simulink model "no_clock_simulink"  (Simulink 7.8)
settings: Solver=VariableStepDiscrete  StartTime=0.0  StopTime=10.0  RelTol=1e-3
values from neighbouring files (symbols this model uses):
  in24b = uut.v_24bit    [no_clock_index_test.m]    (also in no_clock_test.m = double(uut.in_24bit))
  in64b1 = double(typecast(uut.in_64bit,'uint32'))    [no_clock_test.m]
  in64b2 = 0    [no_clock_test.m]
  in8b = double(uut.in_8bit)    [no_clock_test.m]
  in96b1 = double(typecast(uut.in_96bit(1),'uint32'))    [no_clock_test.m]
  in96b2 = double(typecast(uut.in_96bit(2),'uint32'))    [no_clock_test.m]
  in96b3 = double(typecast(uut.in_96bit(3),'uint32'))    [no_clock_test.m]
settings Model: Creator=chuh  LastModifiedBy=chuh

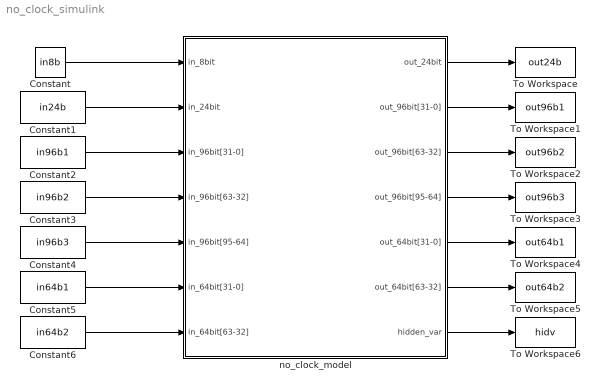
== system no_clock_simulink ==
  Constant : Constant  Value=in8b
  Constant1 : Constant  Value=in24b
  Constant2 : Constant  Value=in96b1
  Constant3 : Constant  Value=in96b2
  Constant4 : Constant  Value=in96b3
  Constant5 : Constant  Value=in64b1
  Constant6 : Constant  Value=in64b2
  To Workspace : ToWorkspace  VariableName=out24b  SampleTime=-1  SaveFormat=Array
  To Workspace1 : ToWorkspace  VariableName=out96b1  SampleTime=-1  SaveFormat=Array
  To Workspace2 : ToWorkspace  VariableName=out96b2  SampleTime=-1  SaveFormat=Array
  To Workspace3 : ToWorkspace  VariableName=out96b3  SampleTime=-1  SaveFormat=Array
  To Workspace4 : ToWorkspace  VariableName=out64b1  SampleTime=-1  SaveFormat=Array
  To Workspace5 : ToWorkspace  VariableName=out64b2  SampleTime=-1  SaveFormat=Array
  To Workspace6 : ToWorkspace  VariableName=hidv  SampleTime=-1  SaveFormat=Array
  no_clock_model : Subsystem  mask(no_clock_model){params_samples=0.001}
      mask prompts: params_samples "Sample time:"
      mask help:
      | input in_8bit[7:0]
      | input in_24bit[23:0]
      | input in_96bit[95:0]
      | input in_64bit[63:0]
      | output out_24bit[23:0]
      | output out_96bit[95:0]
      | output out_64bit[63:0]
      | output hidden_var
      mask Help:
      | input in_8bit[7:0]
      | input in_24bit[23:0]
      | input in_96bit[95:0]
      | input in_64bit[63:0]
      | output out_24bit[23:0]
      | output out_96bit[95:0]
      | output out_64bit[63:0]
      | output hidden_var
  wires:
  Constant/1 -> no_clock_model/1(in_8bit)
  Constant1/1 -> no_clock_model/2(in_24bit)
  Constant2/1 -> no_clock_model/3(in_96bit[31-0])
  Constant3/1 -> no_clock_model/4(in_96bit[63-32])
  Constant4/1 -> no_clock_model/5(in_96bit[95-64])
  Constant5/1 -> no_clock_model/6(in_64bit[31-0])
  Constant6/1 -> no_clock_model/7(in_64bit[63-32])
  no_clock_model/1(out_24bit) -> To Workspace/1
  no_clock_model/2(out_96bit[31-0]) -> To Workspace1/1
  no_clock_model/3(out_96bit[63-32]) -> To Workspace2/1
  no_clock_model/4(out_96bit[95-64]) -> To Workspace3/1
  no_clock_model/5(out_64bit[31-0]) -> To Workspace4/1
  no_clock_model/6(out_64bit[63-32]) -> To Workspace5/1
  no_clock_model/7(hidden_var) -> To Workspace6/1

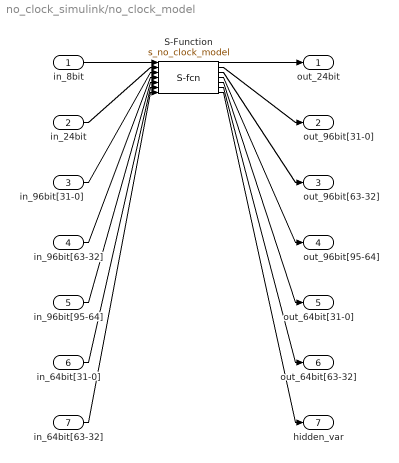
== system no_clock_simulink/no_clock_model ==
  in_8bit : Inport  OutDataTypeStr=double  SampleTime=0.001
  in_24bit : Inport  Port=2  OutDataTypeStr=double  SampleTime=0.001
  in_96bit[31-0] : Inport  Port=3  OutDataTypeStr=double  SampleTime=0.001
  in_96bit[63-32] : Inport  Port=4  OutDataTypeStr=double  SampleTime=0.001
  in_96bit[95-64] : Inport  Port=5  OutDataTypeStr=double  SampleTime=0.001
  in_64bit[31-0] : Inport  Port=6  OutDataTypeStr=double  SampleTime=0.001
  in_64bit[63-32] : Inport  Port=7  OutDataTypeStr=double  SampleTime=0.001
  S-Function : S-Function  FunctionName=s_no_clock_model  Parameters=params_samples  EnableBusSupport=off
  out_24bit : Outport  OutDataTypeStr=uint32  SampleTime=0.001
  out_96bit[31-0] : Outport  Port=2  OutDataTypeStr=uint32  SampleTime=0.001
  out_96bit[63-32] : Outport  Port=3  OutDataTypeStr=uint32  SampleTime=0.001
  out_96bit[95-64] : Outport  Port=4  OutDataTypeStr=uint32  SampleTime=0.001
  out_64bit[31-0] : Outport  Port=5  OutDataTypeStr=uint32  SampleTime=0.001
  out_64bit[63-32] : Outport  Port=6  OutDataTypeStr=uint32  SampleTime=0.001
  hidden_var : Outport  Port=7  OutDataTypeStr=uint32  SampleTime=0.001
  wires:
  in_8bit/1 -> S-Function/1
  in_24bit/1 -> S-Function/2
  in_96bit[31-0]/1 -> S-Function/3
  in_96bit[63-32]/1 -> S-Function/4
  in_96bit[95-64]/1 -> S-Function/5
  in_64bit[31-0]/1 -> S-Function/6
  in_64bit[63-32]/1 -> S-Function/7
  S-Function/1 -> out_24bit/1
  S-Function/2 -> out_96bit[31-0]/1
  S-Function/3 -> out_96bit[63-32]/1
  S-Function/4 -> out_96bit[95-64]/1
  S-Function/5 -> out_64bit[31-0]/1
  S-Function/6 -> out_64bit[63-32]/1
  S-Function/7 -> hidden_var/1
